simulink model "Class6_quiz_Simulink2_Solution"  (R2021a)
settings: Solver=VariableStepAuto  StartTime=0.0  StopTime=10  RelTol=1e-3
settings Model: Creator=Rashedul Islam  LastModifiedBy=Rashedul Islam

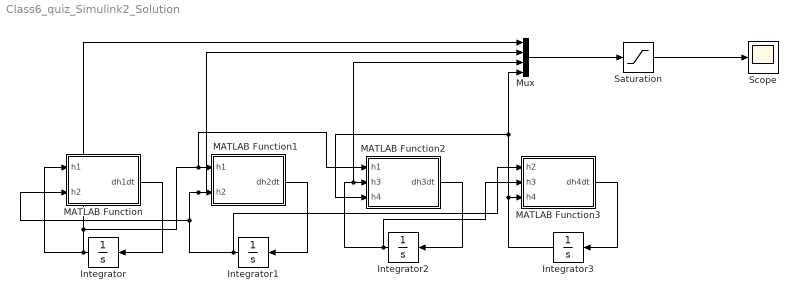
== system Class6_quiz_Simulink2_Solution ==
  Integrator{,1..3} (4 alike) : Integrator
  MATLAB Function : MATLAB Function  TreatAsAtomicUnit=on
  MATLAB Function1 : MATLAB Function  TreatAsAtomicUnit=on
  MATLAB Function2 : MATLAB Function  TreatAsAtomicUnit=on
  MATLAB Function3 : MATLAB Function  TreatAsAtomicUnit=on
  Mux : Mux
  Saturation : Saturate  UpperLimit=6  LowerLimit=0
  Scope : Scope
  wires:
  MATLAB Function/1(dh1dt) -> Integrator/1
  Integrator/1 -> Mux/1, MATLAB Function2/1(h1), MATLAB Function1/1(h1), MATLAB Function/1(h1)
  MATLAB Function1/1(dh2dt) -> Integrator1/1
  Integrator1/1 -> MATLAB Function3/1(h2), Mux/2, MATLAB Function1/2(h2), MATLAB Function/2(h2)
  MATLAB Function2/1(dh3dt) -> Integrator2/1
  Integrator2/1 -> MATLAB Function3/2(h3), Mux/3, MATLAB Function2/2(h3)
  MATLAB Function3/1(dh4dt) -> Integrator3/1
  Integrator3/1 -> Mux/4, MATLAB Function2/3(h4), MATLAB Function3/3(h4)
  Mux/1 -> Saturation/1
  Saturation/1 -> Scope/1

== matlab function Class6_quiz_Simulink2_Solution/MATLAB Function ==
  data: h1 input; dh1dt output; h2 input
function dh1dt = fcn(h1,h2)
q1in=15
q1hout=2.5*(h1-h2)
q1vout=5*h1
A=(pi*.566^2)/4
dh1dt = (q1in-q1hout-q1vout)/A;

== matlab function Class6_quiz_Simulink2_Solution/MATLAB Function2 ==
  data: h1 input; dh3dt output; h3 input; h4 input
function dh3dt = fcn(h1,h3,h4)

q1vout=5*h1
q3hout=2.5*(h3-h4)
A=(pi*.566^2)/4
dh3dt = (q1vout-q3hout)/A;

== matlab function Class6_quiz_Simulink2_Solution/MATLAB Function3 ==
  data: h2 input; h3 input; dh4dt output; h4 input
function dh4dt = fcn(h2,h3,h4)

q3hout=2.5*(h3-h4)
q2vout=5*h2
q4hout=2.5*h4
A=(pi*.566^2)/4
dh4dt = (q3hout+q2vout-q4hout)/A;

== matlab function Class6_quiz_Simulink2_Solution/MATLAB Function1 ==
  data: h1 input; dh2dt output; h2 input
function dh2dt = fcn(h1,h2)
q2in=10
q1hout=2.5*(h1-h2)
q2vout=5*h2
A=(pi*.566^2)/4
dh2dt = (q2in+q1hout-q2vout)/A;
